simulink model "dc_new_1"  (R2016a)
settings: Solver=FixedStepAuto  StartTime=0.0  StopTime=10.0  RelTol=1e-3
undefined symbols (not defined in the file or in its folder): DiscIntNeverNeededParam
libraries: simulink x1, fuzblock x1, cstblocks x1
settings Model: Creator=Admin  LastModifiedBy=Admin

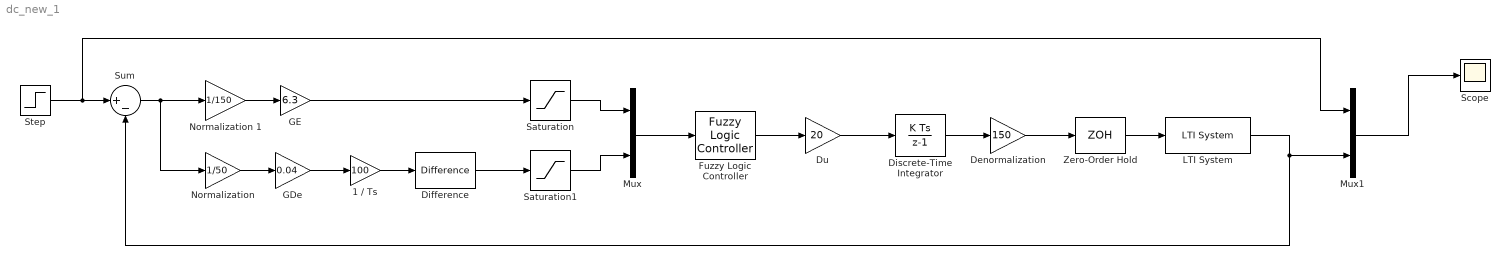
== system dc_new_1 ==
  1 / Ts : Gain  Gain=100
  Denormalization : Gain  Gain=150
  Difference : simulink/Discrete/Difference  ICPrevInput=0.0  OutMin=[]  OutMax=[]  OutDataType=fixdt(1, 16)  OutScaling=2^-10  DoSatur=off
  Discrete-Time Integrator : DiscreteIntegrator  InitialConditionSetting=State (most efficient)  SampleTime=0.01  ICPrevOutput=DiscIntNeverNeededParam  ICPrevScaledInput=DiscIntNeverNeededParam
  Du : Gain  Gain=20
  Fuzzy Logic Controller : fuzblock/Fuzzy Logic  Controller  fis=['model.fis']
  GDe : Gain  Gain=0.04
  GE : Gain  Gain=6.3
  LTI System : cstblocks/LTI System  sys=tf(18.69,[1 12.064])  IC=[]
  Mux : Mux  Inputs=2
  Mux1 : Mux  Inputs=2
  Normalization : Gain  Gain=1/50
  Normalization 1 : Gain  Gain=1/150
  Saturation : Saturate  UpperLimit=1  LowerLimit=-1
  Saturation1 : Saturate  UpperLimit=1  LowerLimit=-1
  Scope : Scope
  Step : Step  Time=0  After=150  SampleTime=0.01
  Sum : Sum  Inputs=|+-
  Zero-Order Hold : ZeroOrderHold  SampleTime=0.01
  wires:
  Sum/1 -> Normalization/1, Normalization 1/1
  Normalization 1/1 -> GE/1
  Normalization/1 -> GDe/1
  GDe/1 -> 1 / Ts/1
  1 / Ts/1 -> Difference/1
  Difference/1 -> Saturation1/1
  GE/1 -> Saturation/1
  Saturation/1 -> Mux/1
  Saturation1/1 -> Mux/2
  Mux/1 -> Fuzzy Logic Controller/1
  Fuzzy Logic Controller/1 -> Du/1
  Du/1 -> Discrete-Time Integrator/1
  Discrete-Time Integrator/1 -> Denormalization/1
  Denormalization/1 -> Zero-Order Hold/1
  Zero-Order Hold/1 -> LTI System/1
  LTI System/1 -> Mux1/2, Sum/2
  Mux1/1 -> Scope/1
  Step/1 -> Mux1/1, Sum/1
